simulink model "Outer_Tensor_Ex2"  (R2025a)
settings: Solver=VariableStepAuto  StartTime=0.0  StopTime=1000  RelTol=1e-3
undefined symbols (not defined in the file): Correlation_ValidMode, DUT, L, vsva1596, xcvc1702
libraries: aieUtilities x2, aieDSP x1, vmcUtilities x1
settings Model: Creator=sdegala  LastModifiedBy=sdegala
settings ModelReferenceCC: EnableRefExpFcnMdlSchedulingChecks=on
settings RTWCC: GPUComputeCapability=3.5

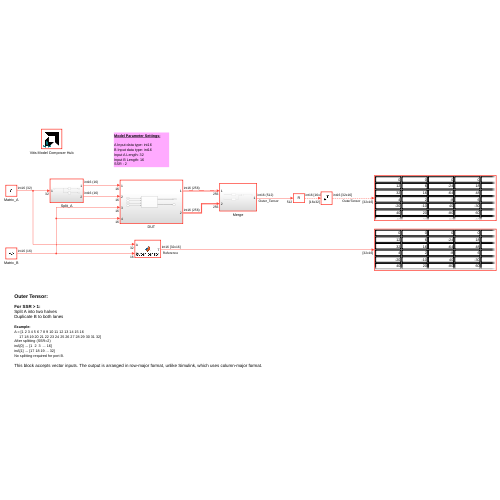
[thumbnail: Simulink's stored preview of the top-level diagram]
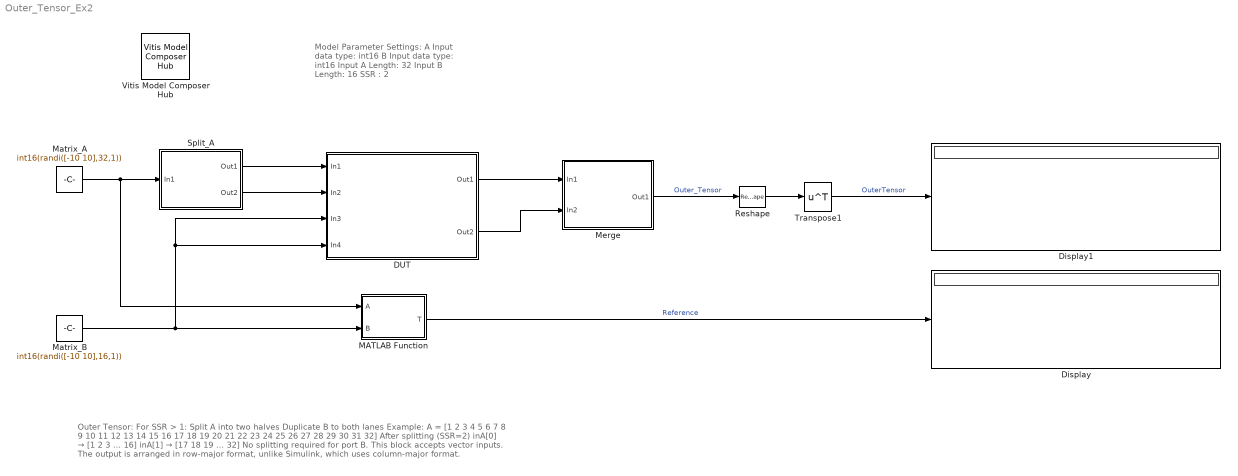
== system Outer_Tensor_Ex2 ==
  note: Outer Tensor:
      |
      | For SSR > 1:
      | Split A into two halves
      | Duplicate B to both lanes
      |
      | Example:
      | A = [1 2 3 4 5 6 7 8 9 10 11 12 13 14 15 16
      | 17 18 19 20 21 22 23 24 25 26 27 28 29 30 31 32]
      | After splitting (SSR=2)
      | inA[0] → [1 2 3 ... 16]
      | inA[1] → [17 18 19 ... 32]
      | No splitting required for port B.
      |
      | This block accepts vector inputs. The output is arranged in row-major format, unlike Simulink, which uses column-major format.
  note: Model Parameter Settings:
      |
      | A Input data type: int16
      | B Input data type: int16
      | Input A Length: 32
      | Input B Length: 16
      | SSR : 2
  DUT : Subsystem
  Display : Display
  Display1 : Display
  MATLAB Function : MATLAB Function  TreatAsAtomicUnit=on
  Matrix_A : Constant  Value=int16(randi([-10 10],32,1))  OutDataTypeStr=int16  SampleTime=1
  Matrix_B : Constant  Value=int16(randi([-10 10],16,1))  OutDataTypeStr=int16  SampleTime=1
  Merge : Subsystem
  Reshape : Reshape  OutputDimensionality=Customize  OutputDimensions=[16,32]
  Split_A : Subsystem
  Transpose1 : Math  Operator=transpose
  Vitis Model Composer Hub : vmcUtilities/Vitis Model Composer Hub  Tag=genX  CodeGeneration=off  SubsystemName=DUT  BlockHierPath=Correlation_ValidMode/DUT  SubsystemType=AIENode  StartColumn=1  NumberOfColumns=1  TargetDirectory=./code  exportDesign=off  analyzeDesign=on  validateDesignOnHw=off  ExportType=AI Engines  IpVendor=xilinx.com  IpLibrary=hls  IpVersion=1.0  IpHWLanguage=Verilog  AieCompilerOptions={}  AieSimulatorOptions={}  CreateTestbench=on  TestbenchStackSize=10  RunRtlSim=off  RunCSim=off  RunAieSim=off  AieSimTimeout=50000  RunAieSimProfiling=off  LaunchVitisAnalyzer=off  PlotOutput=off  RunX86Sim=off  X86SimTimeout=10  GenHwImage=off  GenLibadfXo=off  GenHwValidationCode=off  PlatformType=Not Specified  HwSystemType=Baremetal  HwValidationTarget=hw  ProjDevice=xcvc1702-vsva1596-2LP-e-L  ProjDevicePart=xcvc1702-vsva1596-2LP-e-L  AIEType=AIE  SamplePeriod=-1  ClockFrequency=200  DataPathParallelism=1  xilinxfamily=versalaicore  part=xcvc1702  speed=-2LP-e-L  package=vsva1596  directory=./netlist  testbench=off  incr_netlist=off  synthesis_tool=Vivado  clock_wrapper=Clock Enables  dbl_ovrd=According to Block Masks  dcm_input_clock_period=10  sysclk_period=10  simulink_period=1  eval_field=0  IPInfoJsonString="{\"DUTSubsystemName\":\"DUT\",\"AIESubsystem\":{\"SubsystemName\":\"DUT\",\"TargetDirectory\":\"./code\",\"AIEArrayConfig\":\"Use entire AIE array\",\"StartColumn\":\"0\",\"NumberOfColumns\":\"1\"},\"SubsystemTag\":\"AIENode\"}"  LogFileName=/proj/xhdhdstaff5/sdegala/Head1/HEAD/2025_2_work/AIE_BLOCKS_2025_2/code/model_composer.log  NThreads=4  IPConfigFile=/tmp/vmctmp-11198269997411262707/Correlation_ValidMode_ipconfig.json
  wires:
  DUT/1(Out1) -> Merge/1(In1)
  Matrix_B/1 -> DUT/4(In4), DUT/3(In3), MATLAB Function/2(B)
  MATLAB Function/1(T) -> Display/1  "Reference"
  Matrix_A/1 -> Split_A/1(In1), MATLAB Function/1(A)
  Split_A/1(Out1) -> DUT/1(In1)
  Split_A/2(Out2) -> DUT/2(In2)
  DUT/2(Out2) -> Merge/2(In2)
  Merge/1(Out1) -> Reshape/1  "Outer_Tensor"
  Reshape/1 -> Transpose1/1
  Transpose1/1 -> Display1/1  "OuterTensor"

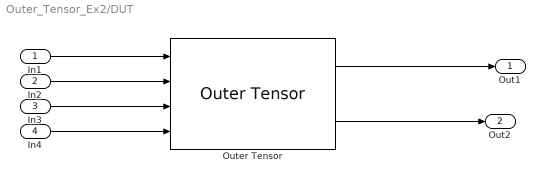
== system Outer_Tensor_Ex2/DUT ==
  In1 : Inport
  In2 : Inport  Port=2
  In3 : Inport  Port=3
  In4 : Inport  Port=4
  Outer Tensor : aieDSP/Outer Tensor  AIE_VARIANT=1  TP_API=0  data_type_A=int16  data_type_B=int16  dim_a=32  dim_b=16  num_frames=1  shift_output=0  ssr=2  rnd_mode=Floor  sat_mode=None  blockJsonConstraints=[]  blockJsonConstraintsInternal=[]  spec=vmc_outer_tensor.json  SerializedMaskParamNames=[]  SerializedMaskParamValues=[]  SerializedMaskParamVisibilities=[]  block_type=Outer Tensor  SerializedMaskParamDataypes=uint|uint|typename|typename|uint|uint|uint|uint|uint|uint|uint  SerializedMaskParamEnumStrArr=0|0|0|0|0|0|0|0|0|Floor,Ceiling,Round to positive infinity,Round to negative infinity,Round symmetrical to infinity,Round symmetrical to zero,Round convergent to even,Round convergent to odd|None,Saturate,Symmetric  SerializedMaskParamEnumValArr=0|0|0|0|0|0|0|0|0|0,1,2,3,4,5,6,7|0,1,3  SerializedMaskParamVectorArr=0|0|0|0|0|0|0|0|0|0|0  SerializedMaskParamKeys=AIE_VARIANT|TP_API|TT_DATA_A|TT_DATA_B|TP_DIM_A|TP_DIM_B|TP_NUM_FRAMES|TP_SHIFT|TP_SSR|TP_RND|TP_SAT
  Out1 : Outport
  Out2 : Outport  Port=2
  wires:
  In2/1 -> Outer Tensor/2
  In1/1 -> Outer Tensor/1
  Outer Tensor/1 -> Out1/1
  In4/1 -> Outer Tensor/4
  In3/1 -> Outer Tensor/3
  Outer Tensor/2 -> Out2/1

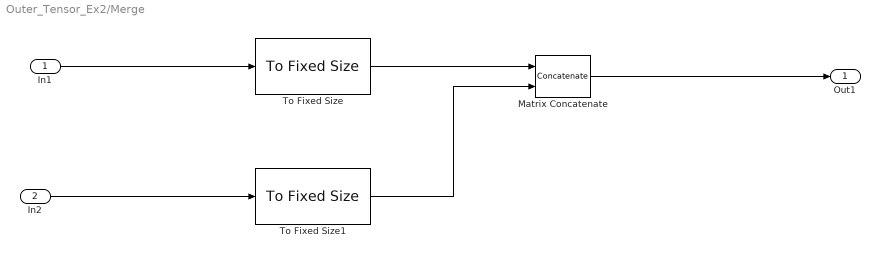
== system Outer_Tensor_Ex2/Merge ==
  In1 : Inport
  In2 : Inport  Port=2
  Matrix Concatenate : Concatenate  ConcatenateDimension=2
  To Fixed Size : aieUtilities/To Fixed Size  Mode=Stop simulation when input variable-size signal is not full  OutputSize=Inherit: Same as input  CopyMethod=Buffer samples to form output  HasStatusOutput=on
  To Fixed Size1 : aieUtilities/To Fixed Size  Mode=Stop simulation when input variable-size signal is not full  OutputSize=Inherit: Same as input  CopyMethod=Buffer samples to form output  HasStatusOutput=on
  Out1 : Outport
  wires:
  In1/1 -> To Fixed Size/1
  In2/1 -> To Fixed Size1/1
  To Fixed Size/1 -> Matrix Concatenate/1
  To Fixed Size1/1 -> Matrix Concatenate/2
  Matrix Concatenate/1 -> Out1/1

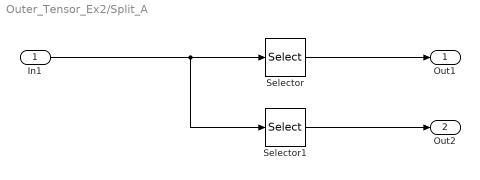
== system Outer_Tensor_Ex2/Split_A ==
  In1 : Inport
  Selector : Selector  InputPortWidth=32  IndexOptions=Index vector (dialog)  Indices=1:1:16  OutputSizes=1
  Selector1 : Selector  InputPortWidth=32  IndexOptions=Index vector (dialog)  Indices=17:1:32  OutputSizes=1
  Out1 : Outport
  Out2 : Outport  Port=2
  wires:
  In1/1 -> Selector/1, Selector1/1
  Selector1/1 -> Out2/1
  Selector/1 -> Out1/1

== matlab function Outer_Tensor_Ex2/MATLAB Function ==
  data: A input; T output; B input
function T = outer_tensor(A, B)
    szA = 32;
    szB = 16;

    Aexp = reshape(A, [szA ones(1,numel(szB))]);
    Bexp = reshape(B, [ones(1,numel(szA)) szB]);

    T = Aexp .* Bexp;
end
